simulink model "DFADAS2_SenFus_v1_201204RC_training_210115"  (R2018b)
settings: Solver=FixedStepDiscrete  StartTime=0.0  StopTime=inf  FixedStep=0.002  RelTol=1e-3  EnableMultiTasking=on
PreLoadFcn:
  | RTWConfigurationCB('preloadfcn', bdroot);
libraries: canmsglib x108, simulink x48, canfdmsglib x12
(part 1 of 28)
CloseFcn:
  | rtwprivate ssgencode ModelCloseRequest test
settings Model: Creator=zhang.jianwei  LastModifiedBy=VCDC-Z21
settings DataIOCC: LimitDataPoints=on  SaveFormat=Array
settings OptimizationCC: DefaultParameterBehavior=Inlined  EnhancedBackFolding=on  PassReuseOutputArgsAs=Individual arguments  ExpressionDepthLimit=2147483647  MaxStackSize=64  OptimizeBlockOrder=speed  DifferentSizesBufferReuse=on  OptimizationCustomize=off
settings DebuggingCC: SaveWithParameterizedLinksMsg=none  UnderspecifiedInitializationDetection=Classic  MergeDetectMultiDrivingBlocksExec=none  SignalResolutionControl=TryResolveAllWithWarning  SolverPrmCheckMsg=warning  MultiTaskDSMMsg=warning  MultiTaskCondExecSysMsg=none  ParameterTunabilityLossMsg=error  FcnCallInpInsideContextMsg=warning  StateNameClashWarn=warning  SFUnexpectedBacktrackingDiag=warning  SFNoUnconditionalDefaultTransitionDiag=warning  SFExecutionAtInitializationDiag=none
settings HardwareCC: ProdBitPerPointer=32  ProdBitPerSizeT=32  ProdBitPerPtrDiffT=32  ProdLargestAtomicFloat=None  ProdWordSize=32  ProdHWDeviceType=Infineon->TriCore
settings ModelReferenceCC: PropagateSignalLabelsOutOfModel=off
settings SFSimCC: SimUseLocalCustomCode=off  MATLABDynamicMemAlloc=off
settings RTWCC: SystemTargetFile=hc12.tlc  GenCodeOnly=on  GenerateMakefile=off  TemplateMakefile=hc12_default_tmf  Description=Embedded Target for Motorola HC12 and CodeWarrior (real-time)  GenerateReport=on  RetainRTWFile=on  RTWUseLocalCustomCode=off  Toolchain=Catkin  IncludeHyperlinkInReport=on  LaunchReport=on  GenerateTraceInfo=on  GenerateTraceReport=on  GenerateTraceReportSl=on  GenerateTraceReportSf=on  GenerateTraceReportEml=on
settings CodeAppCC: ForceParamTrailComments=on  IgnoreCustomStorageClasses=off  OperatorAnnotations=on  SimulinkDataObjDesc=on  SFDataObjDesc=on  CustomSymbolStrType=$N$R$M  InternalIdentifier=Classic
settings STFCustomTargetCC: MultiwordLength=256  ModelReferenceCompliant=off  CombineOutputUpdateFcns=on  ERTCustomFileBanners=on  SupportContinuousTime=off  SupportNonInlinedSFcns=off  RemoveResetFunc=on  SupportVariableSizeSignals=on  MATLABClassNameForMDSCustomization=Simulink.SoftwareTarget.ERTCustomization  SystemTargetFile=hc12.tlc
settings ERTTargetCC: ModelReferenceCompliant=off  ParMdlRefBuildCompliant=off  CompOptLevelCompliant=off  ConcurrentExecutionCompliant=off  SupportVariableSizeSignals=on  ModelStepFunctionPrototypeControlCompliant=off  CPPClassGenCompliant=off  UseToolchainInfoCompliant=off  InlinedParameterPlacement=NonHierarchical  ERTCustomFileTemplate=hc12_file_process.tlc
settings ConfigComp: CovMetricSettings=dw  CovHtmlReporting=on  CovSaveCumulativeToWorkspaceVar=on  CovSaveSingleToWorkspaceVar=on  CovExternalEMLEnable=off  CovSFcnEnable=off

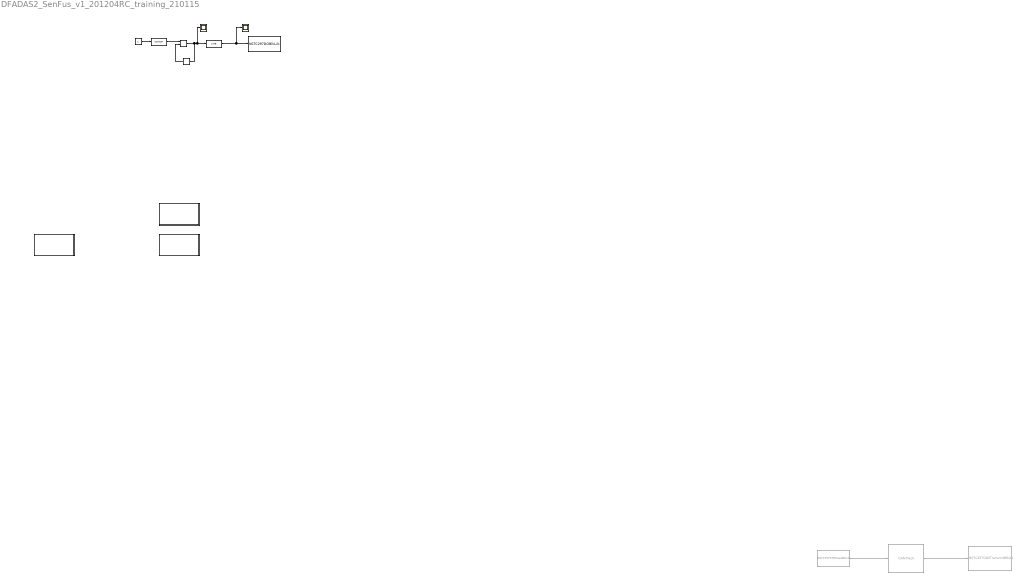
== system DFADAS2_SenFus_v1_201204RC_training_210115 ==
  note: 2ms
  note: Rev.21
      | By VCDC.ASCL.JLU
      | 2020-10-22
  note: iPilot(L3-) Control Software Model
  note: Level: 0
      | Num: 00
      | Rev: 00.00.01
      | Ud: 20-10-26
  CAN Pack11 : canmsglib/CAN Pack  Commented=on  MsgList=(none)  MsgName=CAN Msg  MsgIDType=Standard (11-bit identifier)  MsgIdentifier=138  MsgLength=8  SignalInfo=stm_time$0$32$1$2$1$0$1$0$0$inf$#  NSignals=1  StartBits=str2num('[int32(0)]')  SignalSizes=str2num('[int32(32)]')  ByteOrders=str2num('[int32(1)]')  DataTypes=str2num('[int32(2)]')  MultiplexTypes=str2num('[int32(1)]')  MultiplexValues=str2num('[double(0)]')  Factors=str2num('[double(1)]')  Offsets=str2num('[double(0)]')  Minimums=str2num('[double(0)]')  Maximums=str2num('[double(inf)]')  Remote=off  ApplyMinMax=off  BusOutput=on
      settings: SourceProductName=Simulink Real-Time  SourceProductBaseCode=XP  DataFormat=manually specified signals
  Constant : Constant  SampleTime=1
  Data Type Conversion : DataTypeConversion  OutDataTypeStr=boolean
  Data Type Conversion3 : DataTypeConversion  OutDataTypeStr=uint8
  Logical Operator : Logic  Operator=NAND  AllPortsSameDT=off  OutDataTypeStr=boolean
  Measure Calibration Debug : Subsystem
      mask Display:
      | color('blue');
      | text(0.98,0.9,'iPilot Software Model','horizontalAlignment','right');
      | color('black');
      | text(0.5,0.5,'Measure Calibration Debug(MCD)','horizontalAlignment','center');
      | text(0.5,0.4,'(10ms)','horizontalAlignment','center');
  Memory : Memory  InheritSampleTime=on
  Resource Initialization : Subsystem
      mask Display:
      | color('green');
      | text(0.98,0.9,'iPilot Control Software Model','horizontalAlignment','right');
      | color('green');
      | text(0.5,0.5,'Resource Initialization','horizontalAlignment','center');
  S-Function : S-Function  FunctionName=NSTC297DOBlkLib  Parameters=|  SFunctionDeploymentMode=off  EnableBusSupport=off  mask(NSTC297 DO){Ns_DOPortNum=23, Ns_DOChannelNum=1, Ns_InitialValue=0, Ns_SampleTime=-1}
      | uint16(Ns_DOPortNum),
      | uint16(Ns_DOChannelNum),
      | uint8(Ns_InitialValue),
      | double(Ns_SampleTime)
      mask prompts: Ns_DOPortNum "Port number:"; Ns_DOChannelNum "Channel number:"; Ns_InitialValue "Initial value:"; Ns_SampleTime "Sample time:"
      mask TypeOptions Ns_InitialValue: 0 | 1
      mask Display:
      | color('blue');
      | text(0.98,0.9,'NovSteeds TC297','horizontalAlignment','right');
      | color('black');
      | text(0.5,0.5,'Digital Output','horizontalAlignment','center');
      | port_label('Input',1,'In');
  S-Function14 : S-Function  Commented=on  FunctionName=NSTC297STMReadBlkLib  Parameters=|  SFunctionDeploymentMode=off  EnableBusSupport=off  mask(NSTC297STMRead){Ns_ChannelNum=0, Ns_TimeUnit=s, Ns_SampleTime=0.05}
      | uint16(Ns_ChannelNum),
      | uint16(Ns_TimeUnit),
      | double(Ns_SampleTime)
      mask prompts: Ns_ChannelNum "Channel number:"; Ns_TimeUnit "Time uint:"; Ns_SampleTime "Sample time:"
      mask TypeOptions Ns_ChannelNum: 0 | 1 | 2
      mask TypeOptions Ns_TimeUnit: us | ms | s
      mask Display:
      | color('blue');
      | text(0.98,0.9,'NovSteeds TC297','horizontalAlignment','right');
      | color('black');
      | text(0.5,0.5,'STM Read','horizontalAlignment','center');
      | port_label('Output',1,'Out');
  S-Function15 : S-Function  Commented=on  FunctionName=NSTC297CANTransmitBlkLib  Parameters=|  SFunctionDeploymentMode=off  EnableBusSupport=off  mask(NSTC297 CAN Transmit){Ns_DeviceID=ADAS Control Unit Gen2, Ns_ChannelNum=5, Ns_FrameType=CAN, Ns_FrameBufferSize=0, Ns_OverflowCntOutFlg=off, Ns_SampleTime=-1}
      | uint16(Ns_DeviceID),
      | uint16(Ns_ChannelNum),
      | uint16(Ns_FrameType),
      | uint16(Ns_FrameBufferSize),
      | uint8(Ns_OverflowCntOutFlg),
      | double(Ns_SampleTime)
      mask prompts: Ns_DeviceID "Device:"; Ns_ChannelNum "Channel number:"; Ns_FrameType "Frame type:"; Ns_FrameBufferSize "Frame buffer size:"; Ns_OverflowCntOutFlg "Overflow count output"; Ns_SampleTime "Sample time:"
      mask init:
      | NSTC297CANTransmit_callback('portlabels');
      mask TypeOptions Ns_DeviceID: General Control Unit Gen2 | ADAS Control Unit Gen2
      mask TypeOptions Ns_ChannelNum: 0 | 1 | 2 | 3 | 4 | 5
      mask TypeOptions Ns_FrameType: CAN | CANFD
      mask Display: color('blue');text(0.98,0.9,'NovSteeds TC297','horizontalAlignment','right');color('blue');text(0.5,0.65,'CAN Transmit','horizontalAlignment','center');color('black');text(0.5,0.35,'Type: CAN','horizontalAlignment','center');text(0.5,0.50,'Channel: 5','horizontalAlignment','center');port_label('input',1, 'Msg');
  Scope : Scope
  Scope1 : Scope
  Signal Input (Input) : Subsystem
  wires:
  Data Type Conversion3/1 -> S-Function/1, Scope1/1
  Logical Operator/1 -> Memory/1, Data Type Conversion3/1, Scope/1
  Memory/1 -> Logical Operator/2
  Data Type Conversion/1 -> Logical Operator/1
  Constant/1 -> Data Type Conversion/1
  CAN Pack11/1 -> S-Function15/1
  S-Function14/1 -> CAN Pack11/1

== system DFADAS2_SenFus_v1_201204RC_training_210115/Measure Calibration Debug ==
  CAN Monitor (CANMon) : Subsystem
      mask Display:
      | color('blue');
      | text(0.98,0.9,'iPilot Software Model','horizontalAlignment','right');
      | color('black');
      | text(0.5,0.5,'CAN Monintor(CANMon)','horizontalAlignment','center');
      | text(0.5,0.4,'(10ms)','horizontalAlignment','center');

== system DFADAS2_SenFus_v1_201204RC_training_210115/Resource Initialization ==
  note: TC297 CAN通道使用配置
      | ◆ ch0--监视与下载（ 有终端电阻 ）
      | ◆ ch1-- FL(S2)、 FR(S3)
      | ◆ ch2--RL(S0)、 RR(S1)
      | ◆ ch3--目标物可视化 （ 有终端电阻 ）
      | ◆ ch4--整车
      | ◆ ch5--ADAS
  note: Level: 1
      | Num: 00
      | Rev: 00.00.01
      | Ud: 20-10-26
  S-Function1 : S-Function  FunctionName=NSTC297CANSetupBlkLib  Parameters=|  SFunctionDeploymentMode=off  EnableBusSupport=off  mask(NSTC297 CAN/CANFD Setup){Ns_DeviceID=ADAS Control Unit Gen2, Ns_ChannelNum=5, Ns_FrameFormat=Standard, Ns_FrameType=CAN, Ns_BaudRate=500kbps, Ns_ArbitrationBaudRate=125kbps, Ns_DataBaudRate=1Mbps}
      | uint16(Ns_DeviceID),
      | uint16(Ns_ChannelNum),
      | uint16(Ns_FrameFormat),
      | uint16(Ns_FrameType),
      | uint16(Ns_BaudRate),
      | uint16(Ns_ArbitrationBaudRate),
      | uint16(Ns_DataBaudRate)
      mask prompts: Ns_DeviceID "Device:"; Ns_ChannelNum "Channel number:"; Ns_FrameFormat "Frame format:"; Ns_FrameType "Frame type:"; Ns_BaudRate "Baud rate:"; Ns_ArbitrationBaudRate "Arbitration Baud rate:"; Ns_DataBaudRate "Data Baud rate:"
      mask init:
      | NSTC297CANSetup_callback('portlabels');
      mask TypeOptions Ns_DeviceID: General Control Unit Gen2 | ADAS Control Unit Gen2
      mask TypeOptions Ns_ChannelNum: 0 | 1 | 2 | 3 | 4 | 5
      mask TypeOptions Ns_FrameFormat: Standard | Extended
      mask TypeOptions Ns_FrameType: CAN | CANFD
      mask Callback Ns_FrameType: NSTC297CANSetup_callback('CAN Type Selection');
      mask TypeOptions Ns_BaudRate: 125kbps | 250kbps | 500kbps | 1Mbps
      mask TypeOptions Ns_ArbitrationBaudRate: 125kbps | 250kbps | 500kbps | 1Mbps
      mask TypeOptions Ns_DataBaudRate: 1Mbps | 2Mbps | 5Mbps | 8Mbps
      mask Display: color('blue');text(0.98,0.9,'NovSteeds TC297','horizontalAlignment','right');color('blue');text(0.5,0.7,'CAN/CANFD Setup','horizontalAlignment','center');color('black');text(0.5,0.6,'Channel: 5','horizontalAlignment','center');text(0.5,0.5,'Format: Standard','horizontalAlignment','center');text(0.5,0.4,'Type: CAN','horizontalAlignment','center');text(0.5,0.3,'Baud rate:500kbps','horizontalAlignment','center');
  S-Function13 : S-Function  FunctionName=NSTC297CANSetupBlkLib  Parameters=|  SFunctionDeploymentMode=off  EnableBusSupport=off  mask(NSTC297 CAN/CANFD Setup){Ns_DeviceID=ADAS Control Unit Gen2, Ns_ChannelNum=2, Ns_FrameFormat=Standard, Ns_FrameType=CANFD, Ns_BaudRate=500kbps, Ns_ArbitrationBaudRate=1Mbps, Ns_DataBaudRate=2Mbps}
      | uint16(Ns_DeviceID),
      | uint16(Ns_ChannelNum),
      | uint16(Ns_FrameFormat),
      | uint16(Ns_FrameType),
      | uint16(Ns_BaudRate),
      | uint16(Ns_ArbitrationBaudRate),
      | uint16(Ns_DataBaudRate)
      mask prompts: Ns_DeviceID "Device:"; Ns_ChannelNum "Channel number:"; Ns_FrameFormat "Frame format:"; Ns_FrameType "Frame type:"; Ns_BaudRate "Baud rate:"; Ns_ArbitrationBaudRate "Arbitration Baud rate:"; Ns_DataBaudRate "Data Baud rate:"
      mask init:
      | NSTC297CANSetup_callback('portlabels');
      mask TypeOptions Ns_DeviceID: General Control Unit Gen2 | ADAS Control Unit Gen2
      mask TypeOptions Ns_ChannelNum: 0 | 1 | 2 | 3 | 4 | 5
      mask TypeOptions Ns_FrameFormat: Standard | Extended
      mask TypeOptions Ns_FrameType: CAN | CANFD
      mask Callback Ns_FrameType: NSTC297CANSetup_callback('CAN Type Selection');
      mask TypeOptions Ns_BaudRate: 125kbps | 250kbps | 500kbps | 1Mbps
      mask TypeOptions Ns_ArbitrationBaudRate: 125kbps | 250kbps | 500kbps | 1Mbps
      mask TypeOptions Ns_DataBaudRate: 1Mbps | 2Mbps | 5Mbps | 8Mbps
      mask Display: color('blue');text(0.98,0.9,'NovSteeds TC297','horizontalAlignment','right');color('blue');text(0.5,0.7,'CAN/CANFD Setup','horizontalAlignment','center');color('black');text(0.5,0.6,'Channel: 2','horizontalAlignment','center');text(0.5,0.5,'Format: Standard','horizontalAlignment','center');text(0.5,0.4,'Type: CANFD','horizontalAlignment','center');text(0.5,0.3,'Baud rate:1Mbps+2Mbps','horizontalAlignment','center');
  S-Function2 : S-Function  FunctionName=NSTC297CANSetupBlkLib  Parameters=|  SFunctionDeploymentMode=off  EnableBusSupport=off  mask(NSTC297 CAN/CANFD Setup){Ns_DeviceID=ADAS Control Unit Gen2, Ns_ChannelNum=0, Ns_FrameFormat=Standard, Ns_FrameType=CAN, Ns_BaudRate=500kbps, Ns_ArbitrationBaudRate=125kbps, Ns_DataBaudRate=1Mbps}
      | uint16(Ns_DeviceID),
      | uint16(Ns_ChannelNum),
      | uint16(Ns_FrameFormat),
      | uint16(Ns_FrameType),
      | uint16(Ns_BaudRate),
      | uint16(Ns_ArbitrationBaudRate),
      | uint16(Ns_DataBaudRate)
      mask prompts: Ns_DeviceID "Device:"; Ns_ChannelNum "Channel number:"; Ns_FrameFormat "Frame format:"; Ns_FrameType "Frame type:"; Ns_BaudRate "Baud rate:"; Ns_ArbitrationBaudRate "Arbitration Baud rate:"; Ns_DataBaudRate "Data Baud rate:"
      mask init:
      | NSTC297CANSetup_callback('portlabels');
      mask TypeOptions Ns_DeviceID: General Control Unit Gen2 | ADAS Control Unit Gen2
      mask TypeOptions Ns_ChannelNum: 0 | 1 | 2 | 3 | 4 | 5
      mask TypeOptions Ns_FrameFormat: Standard | Extended
      mask TypeOptions Ns_FrameType: CAN | CANFD
      mask Callback Ns_FrameType: NSTC297CANSetup_callback('CAN Type Selection');
      mask TypeOptions Ns_BaudRate: 125kbps | 250kbps | 500kbps | 1Mbps
      mask TypeOptions Ns_ArbitrationBaudRate: 125kbps | 250kbps | 500kbps | 1Mbps
      mask TypeOptions Ns_DataBaudRate: 1Mbps | 2Mbps | 5Mbps | 8Mbps
      mask Display: color('blue');text(0.98,0.9,'NovSteeds TC297','horizontalAlignment','right');color('blue');text(0.5,0.7,'CAN/CANFD Setup','horizontalAlignment','center');color('black');text(0.5,0.6,'Channel: 0','horizontalAlignment','center');text(0.5,0.5,'Format: Standard','horizontalAlignment','center');text(0.5,0.4,'Type: CAN','horizontalAlignment','center');text(0.5,0.3,'Baud rate:500kbps','horizontalAlignment','center');
  S-Function3 : S-Function  FunctionName=NSTC297CANSetupBlkLib  Parameters=|  SFunctionDeploymentMode=off  EnableBusSupport=off  mask(NSTC297 CAN/CANFD Setup){Ns_DeviceID=ADAS Control Unit Gen2, Ns_ChannelNum=1, Ns_FrameFormat=Standard, Ns_FrameType=CANFD, Ns_BaudRate=500kbps, Ns_ArbitrationBaudRate=1Mbps, Ns_DataBaudRate=2Mbps}
      | uint16(Ns_DeviceID),
      | uint16(Ns_ChannelNum),
      | uint16(Ns_FrameFormat),
      | uint16(Ns_FrameType),
      | uint16(Ns_BaudRate),
      | uint16(Ns_ArbitrationBaudRate),
      | uint16(Ns_DataBaudRate)
      mask prompts: Ns_DeviceID "Device:"; Ns_ChannelNum "Channel number:"; Ns_FrameFormat "Frame format:"; Ns_FrameType "Frame type:"; Ns_BaudRate "Baud rate:"; Ns_ArbitrationBaudRate "Arbitration Baud rate:"; Ns_DataBaudRate "Data Baud rate:"
      mask init:
      | NSTC297CANSetup_callback('portlabels');
      mask TypeOptions Ns_DeviceID: General Control Unit Gen2 | ADAS Control Unit Gen2
      mask TypeOptions Ns_ChannelNum: 0 | 1 | 2 | 3 | 4 | 5
      mask TypeOptions Ns_FrameFormat: Standard | Extended
      mask TypeOptions Ns_FrameType: CAN | CANFD
      mask Callback Ns_FrameType: NSTC297CANSetup_callback('CAN Type Selection');
      mask TypeOptions Ns_BaudRate: 125kbps | 250kbps | 500kbps | 1Mbps
      mask TypeOptions Ns_ArbitrationBaudRate: 125kbps | 250kbps | 500kbps | 1Mbps
      mask TypeOptions Ns_DataBaudRate: 1Mbps | 2Mbps | 5Mbps | 8Mbps
      mask Display: color('blue');text(0.98,0.9,'NovSteeds TC297','horizontalAlignment','right');color('blue');text(0.5,0.7,'CAN/CANFD Setup','horizontalAlignment','center');color('black');text(0.5,0.6,'Channel: 1','horizontalAlignment','center');text(0.5,0.5,'Format: Standard','horizontalAlignment','center');text(0.5,0.4,'Type: CANFD','horizontalAlignment','center');text(0.5,0.3,'Baud rate:1Mbps+2Mbps','horizontalAlignment','center');
  S-Function5 : S-Function  FunctionName=NSTC297CANSetupBlkLib  Parameters=|  SFunctionDeploymentMode=off  EnableBusSupport=off  mask(NSTC297 CAN/CANFD Setup){Ns_DeviceID=ADAS Control Unit Gen2, Ns_ChannelNum=3, Ns_FrameFormat=Standard, Ns_FrameType=CANFD, Ns_BaudRate=500kbps, Ns_ArbitrationBaudRate=1Mbps, Ns_DataBaudRate=2Mbps}
      | uint16(Ns_DeviceID),
      | uint16(Ns_ChannelNum),
      | uint16(Ns_FrameFormat),
      | uint16(Ns_FrameType),
      | uint16(Ns_BaudRate),
      | uint16(Ns_ArbitrationBaudRate),
      | uint16(Ns_DataBaudRate)
      mask prompts: Ns_DeviceID "Device:"; Ns_ChannelNum "Channel number:"; Ns_FrameFormat "Frame format:"; Ns_FrameType "Frame type:"; Ns_BaudRate "Baud rate:"; Ns_ArbitrationBaudRate "Arbitration Baud rate:"; Ns_DataBaudRate "Data Baud rate:"
      mask init:
      | NSTC297CANSetup_callback('portlabels');
      mask TypeOptions Ns_DeviceID: General Control Unit Gen2 | ADAS Control Unit Gen2
      mask TypeOptions Ns_ChannelNum: 0 | 1 | 2 | 3 | 4 | 5
      mask TypeOptions Ns_FrameFormat: Standard | Extended
      mask TypeOptions Ns_FrameType: CAN | CANFD
      mask Callback Ns_FrameType: NSTC297CANSetup_callback('CAN Type Selection');
      mask TypeOptions Ns_BaudRate: 125kbps | 250kbps | 500kbps | 1Mbps
      mask TypeOptions Ns_ArbitrationBaudRate: 125kbps | 250kbps | 500kbps | 1Mbps
      mask TypeOptions Ns_DataBaudRate: 1Mbps | 2Mbps | 5Mbps | 8Mbps
      mask Display: color('blue');text(0.98,0.9,'NovSteeds TC297','horizontalAlignment','right');color('blue');text(0.5,0.7,'CAN/CANFD Setup','horizontalAlignment','center');color('black');text(0.5,0.6,'Channel: 3','horizontalAlignment','center');text(0.5,0.5,'Format: Standard','horizontalAlignment','center');text(0.5,0.4,'Type: CANFD','horizontalAlignment','center');text(0.5,0.3,'Baud rate:1Mbps+2Mbps','horizontalAlignment','center');
  S-Function7 : S-Function  FunctionName=NSTC297CANSetupBlkLib  Parameters=|  SFunctionDeploymentMode=off  EnableBusSupport=off  mask(NSTC297 CAN/CANFD Setup){Ns_DeviceID=ADAS Control Unit Gen2, Ns_ChannelNum=4, Ns_FrameFormat=Standard, Ns_FrameType=CAN, Ns_BaudRate=500kbps, Ns_ArbitrationBaudRate=125kbps, Ns_DataBaudRate=1Mbps}
      | uint16(Ns_DeviceID),
      | uint16(Ns_ChannelNum),
      | uint16(Ns_FrameFormat),
      | uint16(Ns_FrameType),
      | uint16(Ns_BaudRate),
      | uint16(Ns_ArbitrationBaudRate),
      | uint16(Ns_DataBaudRate)
      mask prompts: Ns_DeviceID "Device:"; Ns_ChannelNum "Channel number:"; Ns_FrameFormat "Frame format:"; Ns_FrameType "Frame type:"; Ns_BaudRate "Baud rate:"; Ns_ArbitrationBaudRate "Arbitration Baud rate:"; Ns_DataBaudRate "Data Baud rate:"
      mask init:
      | NSTC297CANSetup_callback('portlabels');
      mask TypeOptions Ns_DeviceID: General Control Unit Gen2 | ADAS Control Unit Gen2
      mask TypeOptions Ns_ChannelNum: 0 | 1 | 2 | 3 | 4 | 5
      mask TypeOptions Ns_FrameFormat: Standard | Extended
      mask TypeOptions Ns_FrameType: CAN | CANFD
      mask Callback Ns_FrameType: NSTC297CANSetup_callback('CAN Type Selection');
      mask TypeOptions Ns_BaudRate: 125kbps | 250kbps | 500kbps | 1Mbps
      mask TypeOptions Ns_ArbitrationBaudRate: 125kbps | 250kbps | 500kbps | 1Mbps
      mask TypeOptions Ns_DataBaudRate: 1Mbps | 2Mbps | 5Mbps | 8Mbps
      mask Display: color('blue');text(0.98,0.9,'NovSteeds TC297','horizontalAlignment','right');color('blue');text(0.5,0.7,'CAN/CANFD Setup','horizontalAlignment','center');color('black');text(0.5,0.6,'Channel: 4','horizontalAlignment','center');text(0.5,0.5,'Format: Standard','horizontalAlignment','center');text(0.5,0.4,'Type: CAN','horizontalAlignment','center');text(0.5,0.3,'Baud rate:500kbps','horizontalAlignment','center');

== system DFADAS2_SenFus_v1_201204RC_training_210115/Signal Input (Input) ==
  note: Level: 0
      | Num: 00
      | Rev: 00.00.01
      | Ud: 20-10-26
  Bus Creator : BusCreator  Inputs=2
  Signal Input (10ms) (Input10) : Subsystem  TreatAsAtomicUnit=on
  Signal Input (50ms) (Input50) : Subsystem  TreatAsAtomicUnit=on
  tag scope: RawIn_bsInInfo=global
  wires:
  Signal Input (10ms) (Input10)/1(Input_bsRawInfo10) -> Bus Creator/2  "RawIn_bsInInfo10"
  Signal Input (50ms) (Input50)/1(Input_bsRawInfo50) -> Bus Creator/1  "RawIn_bsInInfo50"
  Bus Creator/1 -> [RawIn_bsInInfo]  "RawIn_bsInInfo"

== system DFADAS2_SenFus_v1_201204RC_training_210115/Measure Calibration Debug/CAN Monitor (CANMon) ==
  note: 2000-2031 雷达信息
  note: 2032-2039 融合信息
  Bus Selector : BusSelector  OutputSignals=RawIn_bsInInfo50.EnvSens.RawObjInfo.RdrFCnr.FLRdr,RawIn_bsInInfo50.EnvSens.RawObjInfo.RdrFCnr.FRRdr,RawIn_bsInInfo50.EnvSens.RawObjInfo.RdrRCnr.RLRdr,RawIn_bsInInfo50.EnvSens.RawObjInfo.RdrRCnr.RRRdr
  Bus Selector1 : BusSelector  Commented=on  OutputSignals=1-10.RLObj1,1-10.RLObj2,1-10.RLObj3,1-10.RLObj4,1-10.RLObj5,1-10.RLObj6,1-10.RLObj7,1-10.RLObj8
  Bus Selector6 : BusSelector  OutputSignals=RawIn_bsInInfo10.bsVehInfo.VehMovRx_bsVehMovInfo.VehMovRx_dphiYawRate,RawIn_bsInInfo10.bsVehInfo.VehMovRx_bsVehMovInfo.VehMovRx_vVehSpd,RawIn_bsInInfo10.bsVehInfo.SWARx_bsSWAInfo.SWARx_phiSWA
  CAN Pack7 : canmsglib/CAN Pack  MsgList=(none)  MsgName=CAN Msg  MsgIDType=Standard (11-bit identifier)  MsgIdentifier=2040  MsgLength=8  SignalInfo=dphi$0$16$1$1$1$0$0.1$0$-Inf$Inf$#V$16$16$1$2$1$0$0.01$0$-Inf$Inf$#phi$32$16$1$1$1$0$0.1$0$-Inf$Inf$#Signal4$48$16$1$2$1$0$1$0$-Inf$Inf$#  NSignals=4  StartBits=str2num('[int32(0);int32(16);int32(32);int32(48)]')  SignalSizes=str2num('[int32(16);int32(16);int32(16);int32(16)]')  ByteOrders=str2num('[int32(1);int32(1);int32(1);int32(1)]')  DataTypes=str2num('[int32(1);int32(2);int32(1);int32(2)]')  MultiplexTypes=str2num('[int32(1);int32(1);int32(1);int32(1)]')  MultiplexValues=str2num('[double(0);double(0);double(0);double(0)]')  Factors=str2num('[double(0.1);double(0.01);double(0.1);double(1)]')  Offsets=str2num('[double(0);double(0);double(0);double(0)]')  Minimums=str2num('[double(-Inf);double(-Inf);double(-Inf);double(-Inf)]')  Maximums=str2num('[double(Inf);double(Inf);double(Inf);double(Inf)]')  Remote=off  ApplyMinMax=off  BusOutput=on
      settings: SourceProductName=Simulink Real-Time  SourceProductBaseCode=XP  DataFormat=manually specified signals
  CamLaneinfo : Subsystem
  CamObjinfo : Subsystem
  FLRdr : Subsystem
  FRRdr : Subsystem
  From : From  Commented=on  GotoTag=FusObjPos  TagVisibility=global
  RLRdr : Subsystem
  RRRdr : Subsystem
  S-Function : S-Function  FunctionName=NSTC297STMReadBlkLib  Parameters=|  SFunctionDeploymentMode=off  EnableBusSupport=off  mask(NSTC297STMRead){Ns_ChannelNum=0, Ns_TimeUnit=s, Ns_SampleTime=0.01}
      | uint16(Ns_ChannelNum),
      | uint16(Ns_TimeUnit),
      | double(Ns_SampleTime)
      mask prompts: Ns_ChannelNum "Channel number:"; Ns_TimeUnit "Time uint:"; Ns_SampleTime "Sample time:"
      mask TypeOptions Ns_ChannelNum: 0 | 1 | 2
      mask TypeOptions Ns_TimeUnit: us | ms | s
      mask Display:
      | color('blue');
      | text(0.98,0.9,'NovSteeds TC297','horizontalAlignment','right');
      | color('black');
      | text(0.5,0.5,'STM Read','horizontalAlignment','center');
      | port_label('Output',1,'Out');
  S-Function6 : S-Function  FunctionName=NSTC297CANTransmitBlkLib  Parameters=|  SFunctionDeploymentMode=off  EnableBusSupport=off  mask(NSTC297 CAN Transmit){Ns_DeviceID=General Control Unit Gen2, Ns_ChannelNum=0, Ns_FrameType=CAN, Ns_FrameBufferSize=0, Ns_OverflowCntOutFlg=off, Ns_SampleTime=-1}
      | uint16(Ns_DeviceID),
      | uint16(Ns_ChannelNum),
      | uint16(Ns_FrameType),
      | uint16(Ns_FrameBufferSize),
      | uint8(Ns_OverflowCntOutFlg),
      | double(Ns_SampleTime)
      mask prompts: Ns_DeviceID "Device:"; Ns_ChannelNum "Channel number:"; Ns_FrameType "Frame type:"; Ns_FrameBufferSize "Frame buffer size:"; Ns_OverflowCntOutFlg "Overflow count output"; Ns_SampleTime "Sample time:"
      mask init:
      | NSTC297CANTransmit_callback('portlabels');
      mask TypeOptions Ns_DeviceID: General Control Unit Gen2 | ADAS Control Unit Gen2
      mask TypeOptions Ns_ChannelNum: 0 | 1 | 2 | 3 | 4 | 5
      mask TypeOptions Ns_FrameType: CAN | CANFD
      mask Display: color('blue');text(0.98,0.9,'NovSteeds TC297','horizontalAlignment','right');color('blue');text(0.5,0.65,'CAN Transmit','horizontalAlignment','center');color('black');text(0.5,0.35,'Type: CAN','horizontalAlignment','center');text(0.5,0.50,'Channel: 0','horizontalAlignment','center');port_label('input',1, 'Msg');
  Subsystem : Subsystem  Commented=on
  Subsystem1 : Subsystem  Commented=on
  Subsystem2 : Subsystem  Commented=on
  Subsystem3 : Subsystem  Commented=on
  Subsystem4 : Subsystem  Commented=on
  Subsystem5 : Subsystem  Commented=on
  Subsystem6 : Subsystem  Commented=on
  Subsystem7 : Subsystem  Commented=on
  wires:
  From/1 -> Bus Selector1/1
  [RawIn_bsInInfo] -> CamObjinfo/1(In1), CamLaneinfo/1(In1), Bus Selector/1
  Bus Selector/1 -> FLRdr/1(<FLRdr>)  "<FLRdr>"
  Bus Selector/2 -> FRRdr/1(<FRRdr>)  "<FRRdr>"
  Bus Selector/3 -> RLRdr/1(<RLRdr>)  "<RLRdr>"
  Bus Selector/4 -> RRRdr/1(<RRRdr>)  "<RRRdr>"
  Bus Selector1/1 -> Subsystem/1(<RLObj1>)  "<RLObj1>"
  Bus Selector1/2 -> Subsystem1/1(<RLObj2>)  "<RLObj2>"
  Bus Selector1/4 -> Subsystem3/1(<RLObj4>)  "<RLObj4>"
  Bus Selector1/3 -> Subsystem2/1(<RLObj3>)  "<RLObj3>"
  Bus Selector1/7 -> Subsystem6/1(<RLObj7>)  "<RLObj7>"
  Bus Selector1/8 -> Subsystem7/1(<RLObj8>)  "<RLObj8>"
  Bus Selector1/6 -> Subsystem5/1(<RLObj6>)  "<RLObj6>"
  Bus Selector1/5 -> Subsystem4/1(<RLObj5>)  "<RLObj5>"
  [RawIn_bsInInfo] -> Bus Selector6/1
  CAN Pack7/1 -> S-Function6/1
  Bus Selector6/1 -> CAN Pack7/1  "<VehMovRx_dphiYawRate>"
  Bus Selector6/2 -> CAN Pack7/2  "<VehMovRx_vVehSpd>"
  Bus Selector6/3 -> CAN Pack7/3  "<SWARx_phiSWA>"
  S-Function/1 -> CAN Pack7/4

== system DFADAS2_SenFus_v1_201204RC_training_210115/Signal Input (Input)/Signal Input (10ms) (Input10) ==
  note: Level: 1
      | Num: 00
      | Rev: 00.00.01
      | Ud: 20-10-26
  Bus Creator1 : BusCreator  Inputs=2
  Others : Subsystem
  VehInfo : Subsystem
  Input_bsRawInfo10 : Outport
  wires:
  VehInfo/1(VehInfo) -> Bus Creator1/1  "bsVehInfo"
  Bus Creator1/1 -> Input_bsRawInfo10/1  "Input_bsRawInfo10"
  Others/1(Out1) -> Bus Creator1/2  "bsOthers"

== system DFADAS2_SenFus_v1_201204RC_training_210115/Signal Input (Input)/Signal Input (50ms) (Input50) ==
  note: Level: 1
      | Num: 00
      | Rev: 00.00.01
      | Ud: 20-10-26
  Bus Creator : BusCreator  Inputs=4
  Bus Creator1 : BusCreator  Inputs=2
  Bus Creator2 : BusCreator  Inputs=2
  Bus Creator3 : BusCreator  Inputs=2
  Bus Creator4 : BusCreator  Inputs=3
  Cmr : Subsystem
  Front Left Radar(S2) Objects Information (FLRdr) : Subsystem  Priority=100
  Front Right Radar(S3) Objects Information (FRRdr) : Subsystem  Priority=100
  Others : Subsystem
  RdrFrt : Subsystem
  Rear Left Radar(S0) Objects Information (RLRdr) : Subsystem  Priority=100
  Rear Right Radar(S1) Objects Information (RRRdr) : Subsystem  Priority=100
  Input_bsRawInfo50 : Outport
  wires:
  Front Right Radar(S3) Objects Information (FRRdr)/1(FRRdr_bsObjInfo) -> Bus Creator3/2  "FRRdr"
  Front Left Radar(S2) Objects Information (FLRdr)/1(FLRdr_bsObjInfo) -> Bus Creator3/1  "FLRdr"
  Cmr/3(Cmr_bsObjInfo) -> Bus Creator/1  "CmrFrt"
  RdrFrt/1(Out1) -> Bus Creator/2  "RdrFrt"
  Bus Creator1/1 -> Input_bsRawInfo50/1
  Bus Creator4/1 -> Bus Creator1/1  "EnvSens"
  Bus Creator3/1 -> Bus Creator/3  "RdrFCnr"
  Cmr/1(Cmr_bsComInfo) -> Bus Creator4/1  "RawLaneInfo"
  Bus Creator/1 -> Bus Creator4/3  "RawObjInfo"
  Cmr/2(Cmr_bsTrafSig) -> Bus Creator4/2  "RawTrafSig"
  Others/1(Out1) -> Bus Creator1/2  "Others"
  Bus Creator2/1 -> Bus Creator/4  "RdrRCnr"
  Rear Right Radar(S1) Objects Information (RRRdr)/1(RRRdr_bsObjInfo) -> Bus Creator2/2  "RRRdr"
  Rear Left Radar(S0) Objects Information (RLRdr)/1(RLRdr_bsObjInfo) -> Bus Creator2/1  "RLRdr"

== system DFADAS2_SenFus_v1_201204RC_training_210115/Measure Calibration Debug/CAN Monitor (CANMon)/CamLaneinfo ==
  In1 : Inport
  Bus Selector : BusSelector  OutputSignals=RawIn_bsInInfo50.EnvSens.RawLaneInfo.CmrRxPrcs_bsL0Info,RawIn_bsInInfo50.EnvSens.RawLaneInfo.CmrRxPrcs_bsR0Info,RawIn_bsInInfo50.EnvSens.RawLaneInfo.CmrRxPrcs_bsL1Info,RawIn_bsInInfo50.EnvSens.RawLaneInfo.CmrRxPrcs_bsR1Info
  Bus Selector1 : BusSelector  OutputSignals=CmrRxPrcs_facmL0C0,CmrRxPrcs_facmL0C1,CmrRxPrcs_facmL0C2,CmrRxPrcs_facmL0C3,CmrRxPrcs_facmL0Ql
  Bus Selector2 : BusSelector  OutputSignals=CmrRxPrcs_facmR0C0,CmrRxPrcs_facmR0C1,CmrRxPrcs_facmR0C2,CmrRxPrcs_facmR0C3,CmrRxPrcs_facmR0Ql
  Bus Selector3 : BusSelector  OutputSignals=CmrRxPrcs_facmL1C0,CmrRxPrcs_facmL1C1,CmrRxPrcs_facmL1C2,CmrRxPrcs_facmL1C3,CmrRxPrcs_facmL1Ql
  Bus Selector4 : BusSelector  OutputSignals=CmrRxPrcs_facmR1C0,CmrRxPrcs_facmR1C1,CmrRxPrcs_facmR1C2,CmrRxPrcs_facmR1C3,CmrRxPrcs_facmR1Ql
  CAN Pack3 : canmsglib/CAN Pack  CANdbFile=D:\work\ADAS ECU-Sensor CAN_V2_20190314(1).dbc  MsgList=(none)  MsgName=Video_Lane_Left_A  MsgIDType=Standard (11-bit identifier)  MsgIdentifier=2041  MsgLength=8  SignalInfo=C0_5FA$44$12$2$1$1$0$1.000000e-02$0$-2.048000e+01$2.047000e+01$#C1_5FA$50$10$2$1$1$0$9.765625e-04$0$-3.570000e-01$3.570000e-01$#C2_5FA$24$16$2$1$1$0$1.000000e-06$0$-3.276800e-02$3.276600e-02$#C3_5FA$8$16$2$1$1$0$4.000000e-09$0$-1.310720e-04$1.310680e-04$#Line_Type_5FA$59$3$2$2$1$0$1$0$0$7$#Message_Counter_5FA$48$2$2$2$1$0$1$0$0$3$#Quality_5FA$62$2$2$2$1$0$1$0$0$3$#  NSignals=7  StartBits=str2num('[int32(44);int32(50);int32(24);int32(8);int32(59);int32(48);int32(62)]')  SignalSizes=str2num('[int32(12);int32(10);int32(16);int32(16);int32(3);int32(2);int32(2)]')  ByteOrders=str2num('[int32(2);int32(2);int32(2);int32(2);int32(2);int32(2);int32(2)]')  DataTypes=str2num('[int32(1);int32(1);int32(1);int32(1);int32(2);int32(2);int32(2)]')  MultiplexTypes=str2num('[int32(1);int32(1);int32(1);int32(1);int32(1);int32(1);int32(1)]')  MultiplexValues=str2num('[double(0);double(0);double(0);double(0);double(0);double(0);double(0)]')  Factors=str2num('[double(1.000000e-02);double(9.765625e-04);double(1.000000e-06);double(4.000000e-09);double(1);double(1);double(1)]')  Offsets=str2num('[double(0);double(0);double(0);double(0);double(0);double(0);double(0)]')  Minimums=str2num('[double(-2.048000e+01);double(-3.570000e-01);double(-3.276800e-02);double(-1.310720e-04);double(0);double(0);double(0)]')  Maximums=str2num('[double(2.047000e+01);double(3.570000e-01);double(3.276600e-02);double(1.310680e-04);double(7);double(3);double(3)]')  Remote=off  ApplyMinMax=off  BusOutput=on
      settings: SourceProductName=Simulink Real-Time  SourceProductBaseCode=XP  DataFormat=manually specified signals
  CAN Pack4 : canmsglib/CAN Pack  CANdbFile=D:\work\ADAS ECU-Sensor CAN_V2_20190314(1).dbc  MsgList=(none)  MsgName=Video_Lane_Right_A  MsgIDType=Standard (11-bit identifier)  MsgIdentifier=2042  MsgLength=8  SignalInfo=C0_5FD$44$12$2$1$1$0$1.000000e-02$0$-2.048000e+01$2.047000e+01$#C1_5FD$50$10$2$1$1$0$9.765625e-04$0$-3.570000e-01$3.570000e-01$#C2_5FD$24$16$2$1$1$0$1.000000e-06$0$-3.276800e-02$3.276600e-02$#C3_5FD$8$16$2$1$1$0$4.000000e-09$0$-1.310720e-04$1.310680e-04$#Line_Type_5FD$59$3$2$2$1$0$1$0$0$7$#Message_Counter_5FD$48$2$2$2$1$0$1$0$0$3$#Quality_5FD$62$2$2$2$1$0$1$0$0$3$#  NSignals=7  StartBits=str2num('[int32(44);int32(50);int32(24);int32(8);int32(59);int32(48);int32(62)]')  SignalSizes=str2num('[int32(12);int32(10);int32(16);int32(16);int32(3);int32(2);int32(2)]')  ByteOrders=str2num('[int32(2);int32(2);int32(2);int32(2);int32(2);int32(2);int32(2)]')  DataTypes=str2num('[int32(1);int32(1);int32(1);int32(1);int32(2);int32(2);int32(2)]')  MultiplexTypes=str2num('[int32(1);int32(1);int32(1);int32(1);int32(1);int32(1);int32(1)]')  MultiplexValues=str2num('[double(0);double(0);double(0);double(0);double(0);double(0);double(0)]')  Factors=str2num('[double(1.000000e-02);double(9.765625e-04);double(1.000000e-06);double(4.000000e-09);double(1);double(1);double(1)]')  Offsets=str2num('[double(0);double(0);double(0);double(0);double(0);double(0);double(0)]')  Minimums=str2num('[double(-2.048000e+01);double(-3.570000e-01);double(-3.276800e-02);double(-1.310720e-04);double(0);double(0);double(0)]')  Maximums=str2num('[double(2.047000e+01);double(3.570000e-01);double(3.276600e-02);double(1.310680e-04);double(7);double(3);double(3)]')  Remote=off  ApplyMinMax=off  BusOutput=on
      settings: SourceProductName=Simulink Real-Time  SourceProductBaseCode=XP  DataFormat=manually specified signals
  CAN Pack5 : canmsglib/CAN Pack  CANdbFile=D:\work\ADAS ECU-Sensor CAN_V2_20190314(1).dbc  MsgList=(none)  MsgName=Video_Lane_Next_Left_A  MsgIDType=Standard (11-bit identifier)  MsgIdentifier=2043  MsgLength=8  SignalInfo=C0_5FB$44$12$2$1$1$0$1.000000e-02$0$-2.048000e+01$2.047000e+01$#C1_5FB$50$10$2$1$1$0$9.765625e-04$0$-3.570000e-01$3.570000e-01$#C2_5FB$24$16$2$1$1$0$1.000000e-06$0$-3.276800e-02$3.276600e-02$#C3_5FB$8$16$2$1$1$0$4.000000e-09$0$-1.310720e-04$1.310680e-04$#Line_Type_5FB$59$3$2$2$1$0$1$0$0$7$#Message_Counter_5FB$48$2$2$2$1$0$1$0$0$3$#Quality_5FB$62$2$2$2$1$0$1$0$0$3$#  NSignals=7  StartBits=str2num('[int32(44);int32(50);int32(24);int32(8);int32(59);int32(48);int32(62)]')  SignalSizes=str2num('[int32(12);int32(10);int32(16);int32(16);int32(3);int32(2);int32(2)]')  ByteOrders=str2num('[int32(2);int32(2);int32(2);int32(2);int32(2);int32(2);int32(2)]')  DataTypes=str2num('[int32(1);int32(1);int32(1);int32(1);int32(2);int32(2);int32(2)]')  MultiplexTypes=str2num('[int32(1);int32(1);int32(1);int32(1);int32(1);int32(1);int32(1)]')  MultiplexValues=str2num('[double(0);double(0);double(0);double(0);double(0);double(0);double(0)]')  Factors=str2num('[double(1.000000e-02);double(9.765625e-04);double(1.000000e-06);double(4.000000e-09);double(1);double(1);double(1)]')  Offsets=str2num('[double(0);double(0);double(0);double(0);double(0);double(0);double(0)]')  Minimums=str2num('[double(-2.048000e+01);double(-3.570000e-01);double(-3.276800e-02);double(-1.310720e-04);double(0);double(0);double(0)]')  Maximums=str2num('[double(2.047000e+01);double(3.570000e-01);double(3.276600e-02);double(1.310680e-04);double(7);double(3);double(3)]')  Remote=off  ApplyMinMax=off  BusOutput=on
      settings: SourceProductName=Simulink Real-Time  SourceProductBaseCode=XP  DataFormat=manually specified signals
  CAN Pack6 : canmsglib/CAN Pack  CANdbFile=D:\work\ADAS ECU-Sensor CAN_V2_20190314(1).dbc  MsgList=(none)  MsgName=Video_Lane_Next_Right_A  MsgIDType=Standard (11-bit identifier)  MsgIdentifier=2044  MsgLength=8  SignalInfo=C0_5FE$44$12$2$1$1$0$1.000000e-02$0$-2.048000e+01$2.047000e+01$#C1_5FE$50$10$2$1$1$0$9.765625e-04$0$-3.570000e-01$3.570000e-01$#C2_5FE$24$16$2$1$1$0$1.000000e-06$0$-3.276800e-02$3.276600e-02$#C3_5FE$8$16$2$1$1$0$4.000000e-09$0$-1.310720e-04$1.310680e-04$#Line_Type_5FE$59$3$2$2$1$0$1$0$0$7$#Message_Counter_5FE$48$2$2$2$1$0$1$0$0$3$#Quality_5FE$62$2$2$2$1$0$1$0$0$3$#  NSignals=7  StartBits=str2num('[int32(44);int32(50);int32(24);int32(8);int32(59);int32(48);int32(62)]')  SignalSizes=str2num('[int32(12);int32(10);int32(16);int32(16);int32(3);int32(2);int32(2)]')  ByteOrders=str2num('[int32(2);int32(2);int32(2);int32(2);int32(2);int32(2);int32(2)]')  DataTypes=str2num('[int32(1);int32(1);int32(1);int32(1);int32(2);int32(2);int32(2)]')  MultiplexTypes=str2num('[int32(1);int32(1);int32(1);int32(1);int32(1);int32(1);int32(1)]')  MultiplexValues=str2num('[double(0);double(0);double(0);double(0);double(0);double(0);double(0)]')  Factors=str2num('[double(1.000000e-02);double(9.765625e-04);double(1.000000e-06);double(4.000000e-09);double(1);double(1);double(1)]')  Offsets=str2num('[double(0);double(0);double(0);double(0);double(0);double(0);double(0)]')  Minimums=str2num('[double(-2.048000e+01);double(-3.570000e-01);double(-3.276800e-02);double(-1.310720e-04);double(0);double(0);double(0)]')  Maximums=str2num('[double(2.047000e+01);double(3.570000e-01);double(3.276600e-02);double(1.310680e-04);double(7);double(3);double(3)]')  Remote=off  ApplyMinMax=off  BusOutput=on
      settings: SourceProductName=Simulink Real-Time  SourceProductBaseCode=XP  DataFormat=manually specified signals
  S-Function2 : S-Function  FunctionName=NSTC297CANTransmitBlkLib  Parameters=|  SFunctionDeploymentMode=off  EnableBusSupport=off  mask(NSTC297 CAN Transmit){Ns_DeviceID=General Control Unit Gen2, Ns_ChannelNum=0, Ns_FrameType=CAN, Ns_FrameBufferSize=0, Ns_OverflowCntOutFlg=off, Ns_SampleTime=0.05}
      | uint16(Ns_DeviceID),
      | uint16(Ns_ChannelNum),
      | uint16(Ns_FrameType),
      | uint16(Ns_FrameBufferSize),
      | uint8(Ns_OverflowCntOutFlg),
      | double(Ns_SampleTime)
      mask prompts: Ns_DeviceID "Device:"; Ns_ChannelNum "Channel number:"; Ns_FrameType "Frame type:"; Ns_FrameBufferSize "Frame buffer size:"; Ns_OverflowCntOutFlg "Overflow count output"; Ns_SampleTime "Sample time:"
      mask init:
      | NSTC297CANTransmit_callback('portlabels');
      mask TypeOptions Ns_DeviceID: General Control Unit Gen2 | ADAS Control Unit Gen2
      mask TypeOptions Ns_ChannelNum: 0 | 1 | 2 | 3 | 4 | 5
      mask TypeOptions Ns_FrameType: CAN | CANFD
      mask Display: color('blue');text(0.98,0.9,'NovSteeds TC297','horizontalAlignment','right');color('blue');text(0.5,0.65,'CAN Transmit','horizontalAlignment','center');color('black');text(0.5,0.35,'Type: CAN','horizontalAlignment','center');text(0.5,0.50,'Channel: 0','horizontalAlignment','center');port_label('input',1, 'Msg');
  S-Function3 : S-Function  FunctionName=NSTC297CANTransmitBlkLib  Parameters=|  SFunctionDeploymentMode=off  EnableBusSupport=off  mask(NSTC297 CAN Transmit){Ns_DeviceID=General Control Unit Gen2, Ns_ChannelNum=0, Ns_FrameType=CAN, Ns_FrameBufferSize=0, Ns_OverflowCntOutFlg=off, Ns_SampleTime=0.05}
      | uint16(Ns_DeviceID),
      | uint16(Ns_ChannelNum),
      | uint16(Ns_FrameType),
      | uint16(Ns_FrameBufferSize),
      | uint8(Ns_OverflowCntOutFlg),
      | double(Ns_SampleTime)
      mask prompts: Ns_DeviceID "Device:"; Ns_ChannelNum "Channel number:"; Ns_FrameType "Frame type:"; Ns_FrameBufferSize "Frame buffer size:"; Ns_OverflowCntOutFlg "Overflow count output"; Ns_SampleTime "Sample time:"
      mask init:
      | NSTC297CANTransmit_callback('portlabels');
      mask TypeOptions Ns_DeviceID: General Control Unit Gen2 | ADAS Control Unit Gen2
      mask TypeOptions Ns_ChannelNum: 0 | 1 | 2 | 3 | 4 | 5
      mask TypeOptions Ns_FrameType: CAN | CANFD
      mask Display: color('blue');text(0.98,0.9,'NovSteeds TC297','horizontalAlignment','right');color('blue');text(0.5,0.65,'CAN Transmit','horizontalAlignment','center');color('black');text(0.5,0.35,'Type: CAN','horizontalAlignment','center');text(0.5,0.50,'Channel: 0','horizontalAlignment','center');port_label('input',1, 'Msg');
  S-Function4 : S-Function  FunctionName=NSTC297CANTransmitBlkLib  Parameters=|  SFunctionDeploymentMode=off  EnableBusSupport=off  mask(NSTC297 CAN Transmit){Ns_DeviceID=General Control Unit Gen2, Ns_ChannelNum=0, Ns_FrameType=CAN, Ns_FrameBufferSize=0, Ns_OverflowCntOutFlg=off, Ns_SampleTime=0.05}
      | uint16(Ns_DeviceID),
      | uint16(Ns_ChannelNum),
      | uint16(Ns_FrameType),
      | uint16(Ns_FrameBufferSize),
      | uint8(Ns_OverflowCntOutFlg),
      | double(Ns_SampleTime)
      mask prompts: Ns_DeviceID "Device:"; Ns_ChannelNum "Channel number:"; Ns_FrameType "Frame type:"; Ns_FrameBufferSize "Frame buffer size:"; Ns_OverflowCntOutFlg "Overflow count output"; Ns_SampleTime "Sample time:"
      mask init:
      | NSTC297CANTransmit_callback('portlabels');
      mask TypeOptions Ns_DeviceID: General Control Unit Gen2 | ADAS Control Unit Gen2
      mask TypeOptions Ns_ChannelNum: 0 | 1 | 2 | 3 | 4 | 5
      mask TypeOptions Ns_FrameType: CAN | CANFD
      mask Display: color('blue');text(0.98,0.9,'NovSteeds TC297','horizontalAlignment','right');color('blue');text(0.5,0.65,'CAN Transmit','horizontalAlignment','center');color('black');text(0.5,0.35,'Type: CAN','horizontalAlignment','center');text(0.5,0.50,'Channel: 0','horizontalAlignment','center');port_label('input',1, 'Msg');
  S-Function5 : S-Function  FunctionName=NSTC297CANTransmitBlkLib  Parameters=|  SFunctionDeploymentMode=off  EnableBusSupport=off  mask(NSTC297 CAN Transmit){Ns_DeviceID=General Control Unit Gen2, Ns_ChannelNum=0, Ns_FrameType=CAN, Ns_FrameBufferSize=0, Ns_OverflowCntOutFlg=off, Ns_SampleTime=0.05}
      | uint16(Ns_DeviceID),
      | uint16(Ns_ChannelNum),
      | uint16(Ns_FrameType),
      | uint16(Ns_FrameBufferSize),
      | uint8(Ns_OverflowCntOutFlg),
      | double(Ns_SampleTime)
      mask prompts: Ns_DeviceID "Device:"; Ns_ChannelNum "Channel number:"; Ns_FrameType "Frame type:"; Ns_FrameBufferSize "Frame buffer size:"; Ns_OverflowCntOutFlg "Overflow count output"; Ns_SampleTime "Sample time:"
      mask init:
      | NSTC297CANTransmit_callback('portlabels');
      mask TypeOptions Ns_DeviceID: General Control Unit Gen2 | ADAS Control Unit Gen2
      mask TypeOptions Ns_ChannelNum: 0 | 1 | 2 | 3 | 4 | 5
      mask TypeOptions Ns_FrameType: CAN | CANFD
      mask Display: color('blue');text(0.98,0.9,'NovSteeds TC297','horizontalAlignment','right');color('blue');text(0.5,0.65,'CAN Transmit','horizontalAlignment','center');color('black');text(0.5,0.35,'Type: CAN','horizontalAlignment','center');text(0.5,0.50,'Channel: 0','horizontalAlignment','center');port_label('input',1, 'Msg');
  wires:
  Bus Selector1/4 -> CAN Pack3/4  "<CmrRxPrcs_facmL0C3>"
  Bus Selector1/3 -> CAN Pack3/3  "<CmrRxPrcs_facmL0C2>"
  Bus Selector1/2 -> CAN Pack3/2  "<CmrRxPrcs_facmL0C1>"
  CAN Pack3/1 -> S-Function2/1
  Bus Selector1/5 -> CAN Pack3/7  "<CmrRxPrcs_facmL0Ql>"
  CAN Pack4/1 -> S-Function3/1
  Bus Selector3/4 -> CAN Pack5/4  "<CmrRxPrcs_facmL1C3>"
  Bus Selector3/3 -> CAN Pack5/3  "<CmrRxPrcs_facmL1C2>"
  Bus Selector3/1 -> CAN Pack5/1  "<CmrRxPrcs_facmL1C0>"
  Bus Selector3/2 -> CAN Pack5/2  "<CmrRxPrcs_facmL1C1>"
  CAN Pack5/1 -> S-Function4/1
  Bus Selector3/5 -> CAN Pack5/7  "<CmrRxPrcs_facmL1Ql>"
  Bus Selector4/5 -> CAN Pack6/7  "<CmrRxPrcs_facmR1Ql>"
  CAN Pack6/1 -> S-Function5/1
  Bus Selector4/2 -> CAN Pack6/2  "<CmrRxPrcs_facmR1C1>"
  Bus Selector4/1 -> CAN Pack6/1  "<CmrRxPrcs_facmR1C0>"
  Bus Selector4/3 -> CAN Pack6/3  "<CmrRxPrcs_facmR1C2>"
  Bus Selector4/4 -> CAN Pack6/4  "<CmrRxPrcs_facmR1C3>"
  In1/1 -> Bus Selector/1
  Bus Selector/1 -> Bus Selector1/1  "<CmrRxPrcs_bsL0Info>"
  Bus Selector/2 -> Bus Selector2/1  "<CmrRxPrcs_bsR0Info>"
  Bus Selector/3 -> Bus Selector3/1  "<CmrRxPrcs_bsL1Info>"
  Bus Selector/4 -> Bus Selector4/1  "<CmrRxPrcs_bsR1Info>"
  Bus Selector1/1 -> CAN Pack3/1  "<CmrRxPrcs_facmL0C0>"
  Bus Selector2/1 -> CAN Pack4/1  "<CmrRxPrcs_facmR0C0>"
  Bus Selector2/2 -> CAN Pack4/2  "<CmrRxPrcs_facmR0C1>"
  Bus Selector2/3 -> CAN Pack4/3  "<CmrRxPrcs_facmR0C2>"
  Bus Selector2/4 -> CAN Pack4/4  "<CmrRxPrcs_facmR0C3>"
  Bus Selector2/5 -> CAN Pack4/7  "<CmrRxPrcs_facmR0Ql>"
